simulink model "onda_completa_tri"  (R2024a)
settings: Solver=VariableStepAuto  StartTime=0.0  StopTime=5*1/60  RelTol=1e-3
libraries: nesl_utility x11, fl_lib x10, ee_lib x6
settings Model: Creator=isabelle  LastModifiedBy=pedro
settings RTWCC: GPUComputeCapability=3.5
settings SimscapeCC: SimscapeLogType=all

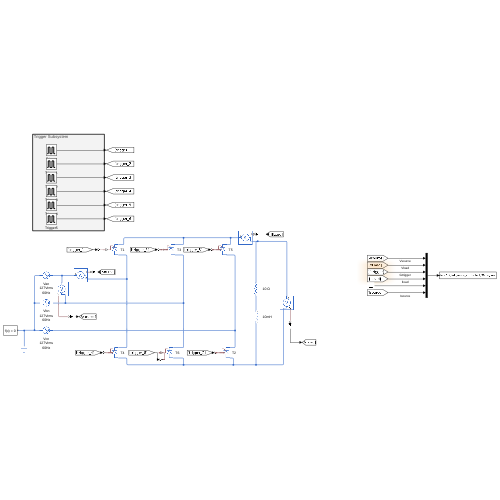
[thumbnail: Simulink's stored preview of the top-level diagram]
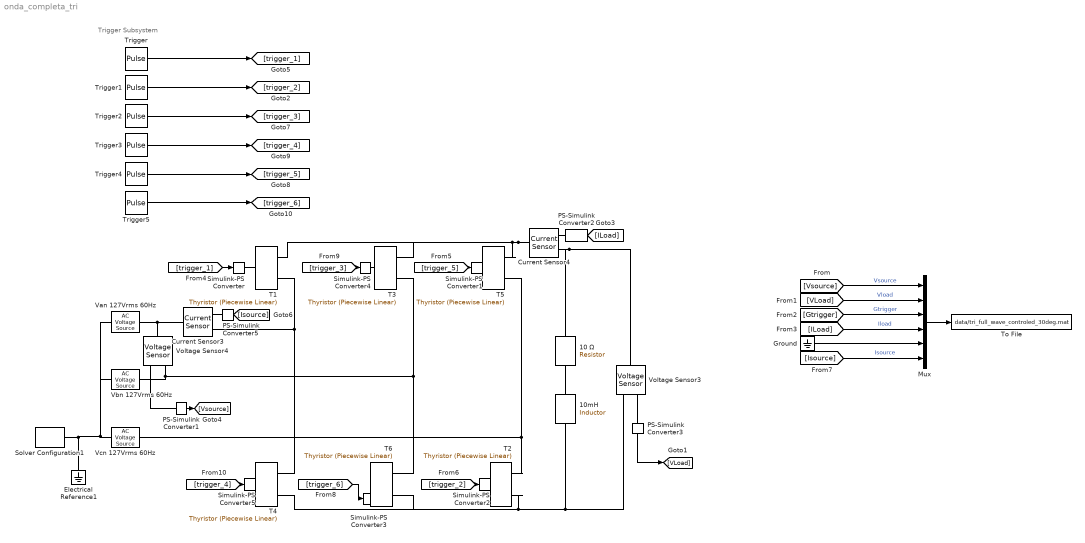
== system onda_completa_tri ==
  note: Trigger Subsystem
  10 Ω : fl_lib/Electrical/Electrical Elements/Resistor  R=10 Ohm  i_specify=off  i_priority=None  i=0 A  i_nominal_specify=off  i_nominal_value=1  i_nominal_unit=A  v_specify=off  v_priority=None  v=0 V  v_nominal_specify=off  v_nominal_value=1  v_nominal_unit=V
  10mH : fl_lib/Electrical/Electrical Elements/Inductor  l=10 mH  r=0 Ohm  g=1e-9 1/Ohm  i_specify=off  i_priority=None  i=0 A  i_nominal_specify=off  i_nominal_value=1  i_nominal_unit=A  v_specify=off  v_priority=None  v=0 V  v_nominal_specify=off  v_nominal_value=1  v_nominal_unit=V  i_L_specify=off  i_L_priority=High  i_L=0 A  i_L_nominal_specify=off  i_L_nominal_value=1  i_L_nominal_unit=A
  Current Sensor3 : fl_lib/Electrical/Electrical Sensors/Current Sensor
  Current Sensor4 : fl_lib/Electrical/Electrical Sensors/Current Sensor
  Electrical Reference1 : fl_lib/Electrical/Electrical Elements/Electrical Reference
  Ground : Ground
  Mux : Mux  Inputs=6
  PS-Simulink Converter{1..3,5} (4 alike) : nesl_utility/PS-Simulink Converter  PhysicalDomain=network_engine_domain  SubClassName=ps_output  LeftPortType=input  RightPortType=output  PseudoPeriodic=off  Frequencies=[]  VectorFormat=inherit  Unit=inherit  AffineConversion=off
  Simulink-PS Converter{,1..5} (6 alike) : nesl_utility/Simulink-PS Converter  PhysicalDomain=network_engine_domain  SubClassName=ps_input  LeftPortType=input  RightPortType=output  PseudoPeriodic=off  Frequencies=[]  NoiseDistribution=none  NoiseParameters=[]  Unit=1  AffineConversion=off  FilteringAndDerivatives=provide  SimscapeFilterOrder=1  InputFilterTimeConstant=0.001  UdotUserProvided=0
  Solver Configuration1 : nesl_utility/Solver Configuration  PhysicalDomain=network_engine_domain  SubClassName=solver  LeftPortType=input  RightPortType=generic  Tones=[]  Harmonics=[]  SimulateNoise=off  Profile=off  UseLocalSampling=off  EnableSwitchedLinearOptims=on  FrequencyDomain=off  UseCCode=off  RelTol=0.001  AbsTol=0.001  MinStep=1e-09  ToWorkspace=off  RevertToSquareIcSolve=off  NumHomotopyIterations=100  PhasorMode=off  PhasorModeNumHarmonics=1  ConsistencySolver=NEWTON_XTOL_AFTER_FTOL  IndexReductionMethod=DerivativeReplacement  DoDC=off  ResidualTolerance=1e-09  ConsistencyTolSource=GLOBAL  ConsistencyAbsTol=0.001  ConsistencyRelTol=0.001  ConsistencyTolFactor=0.001  UseLocalSolver=off  LocalSolverChoice=NE_BACKWARD_EULER_ADVANCER  ResolveIndetEquations=on  FunctionEvalNumThread=1  LocalSolverSampleTime=0.001  DoFixedCost=off  MaxNonlinIter=3  MaxModeIter=2  ComputeImpulses=off  ImpulseIterations=2  LinearAlgebra=auto  LinearAlgebraNumThread=0  EquationFormulation=NE_TIME_EF  DelaysMemoryBudget=1024  AutomaticFiltering=on  FilteringTimeConstant=0.001  PartitionStorageMethod=AS_NEEDED  PartitionMemoryBudget=1024  PartitionMethod=ROBUST  MultibodyUseLocalSolver=off  MultibodyLocalSolverChoice=ODE1  MultibodyLocalSolverSampleTime=0.001
  T{1..6} (6 alike) : ee_lib/Semiconductors & Converters/Thyristor (Piecewise Linear)  port_option=ee.enum.controlport.ps  Vf=1e-6 V  Ron=0.001 Ohm  Goff=1e-5 1/Ohm  Vgt=6 V  Ih=1e-6 A  diode_param=ee.enum.semiconductors.protectionDiode.external  diode_Vf=0.8 V  diode_Ron=0.001 Ohm  diode_Goff=1e-5 1/Ohm  diode_C=50e-9 F  diode_iRM=-235 A  diode_iF=300 A  diode_idot=-50 A/us  diode_trr_param=ee.enum.converters.diodetrr.trr_factor  diode_trr_factor=3  diode_trr=15 us  diode_Qrr=1500 s*uA  iak_specify=off  iak_priority=None  iak=0 A  iak_nominal_specify=off  iak_nominal_value=1  iak_nominal_unit=A  vak_specify=off  vak_priority=None  vak=0 V  vak_nominal_specify=off  vak_nominal_value=1  vak_nominal_unit=V  vgk_specify=off  vgk_priority=None  vgk=0 V  vgk_nominal_specify=off  vgk_nominal_value=1  vgk_nominal_unit=V  thermal_loss_option=ee.enum.converters.thermalLossOption.constantvalues  Von_data=[0, .1, .6, .8, 1, 1.3, 1.6, 2, 2.4; 0, .1, .7, 1, 1.2, 1.5, 1.9, 2.4, 2.8] V  Tj=[298.15, 398.15] K  Iout_data=[0, .1, 1, 5, 10, 20, 40, 70, 100] A  Eon_data=[0, .0024, .024, .12, .2, .48, 1.04, 2.16, 3.24; 0, .003, .03, .15, .25, .6, 1.3, 2.7, 4.05] * 1e-3 J  Tj_loss=[298.15, 398.15] K  Iout_data_loss=[0, .1, 1, 5, 10, 20, 40, 70, 100] A  Eon_scalar=22.86e-3 J  Eoff_natural_commutation=10e-3 J  Voff=300 V  Iout_scalar=600 A  onCurrentMeasDelay=1e-4 s  diodeModelType=ee.enum.converters.diodeModelType.pwl  diodeTableType=ee.enum.diode.tableType.IfMat  diode_IfMat=[.07, .12, .19, 1.75, 4.24, 7.32, 11.2; .16, .3, .72, 2.14, 4.02, 6.35, 9.12] A  diode_VfMat=[.9, 1.15, 1.25, 1.5, 1.75, 2.17, 2.6, 2.85; .58, .68, .75, 1.1, 1.38, 1.77, 2.27, 2.7] V  diode_TjVec=[25, 125] degC  diode_VfVec=[.5, .7, .9, 1.3, 1.7, 2.1, 2.5] V  diode_IfVec=[.1, .2, .5, 1, 2, 4, 7, 10] A  diode_rec_loss_model=ee.enum.diode.reverseRecoveryModel.fixed  diode_ErecVal=0 J  diode_scaleWithIandV=true  diode_ErecMat=zeros(2, 3) J  diode_TjrecVec=[298.15, 398.15] K  diode_IfrecVec=[.1, 1, 10] A  diode_IrecVal=10 A  diode_VrecVal=10 V  diode_tFilter=1 / 1000 / 100 s  thermal_network_parameterization=ee.enum.thermalNetworkTopology.external  Rth=[.08, .5] K/W  Rth_Cauer=[.08, .1, .5] K/W  Rth_Foster=[.08, .14, .22, .16] K/W  thermal_mass_parameterization=ee.enum.thermalNetwork.timeconstant  thermal_mass=[.01, .5] J/K  thermal_mass_Cauer=[.01, .1, .5] J/K  thermal_mass_Foster=[.001, .005, .05, .5] J/K  thermal_time_constant=[.001, .2] s  thermal_time_constant_Cauer=[.001, .1, .2] s  thermal_time_constant_Foster=[7e-05, .0007, .01, .08] s  thermal_mass_initial_temperatures=[25, 25] degC  thermal_mass_initial_temperatures_Cauer=[25, 25, 25] degC  junction_thermal_mass=0.01 J/K  Tvec_initial_Foster=[25, 25, 25, 25] degC  junction_temperature_specify=off  junction_temperature_priority=None  junction_temperature=25 degC  junction_temperature_nominal_specify=off  junction_temperature_nominal_value=1  junction_temperature_nominal_unit=degC  Qj_specify=off  Qj_priority=None  Qj=0 W  Qj_nominal_specify=off  Qj_nominal_value=1  Qj_nominal_unit=W  accumulatedSwitchingLosses_specify=off  accumulatedSwitchingLosses_priority=None  accumulatedSwitchingLosses=0 J
      settings: InternalSimscapePortConfiguration="{\"Bottom\":[],\"Left\":[{\"id\":\"G\",\"label\":\"\",\"type\":\"input\"}],\"Right\":[{\"id\":\"A\",\"label\":\"\",\"type\":\"foundation.electrical.electrical\"},{\"id\":\"K\",\"label\":\"\",\"type\":\"foundation.electrical.electrical\"}],\"Top\":[]}"
  To File : ToFile  Filename=data/tri_full_wave_controled_30deg.mat  SaveFormat=Timeseries
  Trigger : DiscretePulseGenerator  PulseType=Time based  Amplitude=10  Period=1/60  PhaseDelay=(1/(60*2*pi)) * (deg2rad(30+30))
  Trigger1 : DiscretePulseGenerator  PulseType=Time based  Amplitude=10  Period=1/60  PhaseDelay=((1/(60*2*pi)) * (deg2rad(30 +30 + 60)))
  Trigger2 : DiscretePulseGenerator  PulseType=Time based  Amplitude=10  Period=1/60  PhaseDelay=(1/(60*2*pi)) * (deg2rad(30+30+120) )
  Trigger3 : DiscretePulseGenerator  PulseType=Time based  Amplitude=10  Period=1/60  PhaseDelay=(1/(60*2*pi)) * (deg2rad(30+30+180))
  Trigger4 : DiscretePulseGenerator  PulseType=Time based  Amplitude=10  Period=1/60  PhaseDelay=(1/(60*2*pi)) * (deg2rad(30+30+240) )
  Trigger5 : DiscretePulseGenerator  PulseType=Time based  Amplitude=10  Period=1/60  PulseWidth=5  PhaseDelay=(1/(60*2*pi)) * (deg2rad(30+30+300) )
  Van 127Vrms 60Hz : fl_lib/Electrical/Electrical Sources/AC Voltage Source  amp=127*sqrt(2) V  shift=0 deg  frequency=60 Hz
  Vbn 127Vrms 60Hz : fl_lib/Electrical/Electrical Sources/AC Voltage Source  amp=127*sqrt(2) V  shift=-120 deg  frequency=60 Hz
  Vcn 127Vrms 60Hz : fl_lib/Electrical/Electrical Sources/AC Voltage Source  amp=127*sqrt(2) V  shift=120 deg  frequency=60 Hz
  Voltage Sensor3 : fl_lib/Electrical/Electrical Sensors/Voltage Sensor
  Voltage Sensor4 : fl_lib/Electrical/Electrical Sensors/Voltage Sensor
  wires:
  PS-Simulink Converter2/1 -> [ILoad]
  PS-Simulink Converter1/1 -> [Vsource]
  PS-Simulink Converter5/1 -> [Isource]
  PS-Simulink Converter3/1 -> [VLoad]
  Trigger1/1 -> [trigger_2]
  Trigger/1 -> [trigger_1]
  Mux/1 -> To File/1
  Ground/1 -> Mux/5
  [ILoad] -> Mux/4  "Iload"
  [Vsource] -> Mux/1  "Vsource"
  [Isource] -> Mux/6  "Isource"
  [VLoad] -> Mux/2  "Vload"
  [Gtrigger] -> Mux/3  "Gtrigger"
  Trigger2/1 -> [trigger_3]
  [trigger_1] -> Simulink-PS Converter/1
  [trigger_2] -> Simulink-PS Converter2/1
  [trigger_5] -> Simulink-PS Converter1/1
  [trigger_6] -> Simulink-PS Converter3/1
  [trigger_3] -> Simulink-PS Converter4/1
  [trigger_4] -> Simulink-PS Converter5/1
  Trigger3/1 -> [trigger_4]
  Trigger4/1 -> [trigger_5]
  Trigger5/1 -> [trigger_6]
  connections:
  Electrical Reference1/LConn1 -- Solver Configuration1/RConn1 -- Vcn 127Vrms 60Hz/RConn1 -- Vbn 127Vrms 60Hz/RConn1 -- Van 127Vrms 60Hz/RConn1
  Current Sensor3/LConn1 -- Van 127Vrms 60Hz/LConn1 -- Voltage Sensor4/LConn1
  Current Sensor3/RConn2 -- T4/RConn2 -- T1/RConn1
  Voltage Sensor4/RConn2 -- T6/RConn2 -- T3/RConn1 -- Vbn 127Vrms 60Hz/LConn1
  Vcn 127Vrms 60Hz/LConn1 -- T5/RConn1 -- T2/RConn2
  Current Sensor4/LConn1 -- T1/RConn2 -- T3/RConn2 -- T5/RConn2
  Voltage Sensor3/RConn2 -- T4/RConn1 -- T6/RConn1 -- T2/RConn1 -- 10mH/RConn1
  Current Sensor4/RConn2 -- 10 Ω/LConn1 -- Voltage Sensor3/LConn1
  10mH/LConn1 -- 10 Ω/RConn1
  Current Sensor4/RConn1 -- PS-Simulink Converter2/LConn1
  Current Sensor3/RConn1 -- PS-Simulink Converter5/LConn1
  PS-Simulink Converter3/LConn1 -- Voltage Sensor3/RConn1
  PS-Simulink Converter1/LConn1 -- Voltage Sensor4/RConn1
  Simulink-PS Converter/RConn1 -- T1/LConn1
  T2/LConn1 -- Simulink-PS Converter2/RConn1
  T5/LConn1 -- Simulink-PS Converter1/RConn1
  T3/LConn1 -- Simulink-PS Converter4/RConn1
  Simulink-PS Converter5/RConn1 -- T4/LConn1
  Simulink-PS Converter3/RConn1 -- T6/LConn1
